simulink model "cosine_pow4"  (R2021b)
settings: Solver=VariableStepAuto  StartTime=0.0  StopTime=1  RelTol=1e-3
libraries: dspsrcs4 x1
settings Model: Creator=baggo  LastModifiedBy=baggo

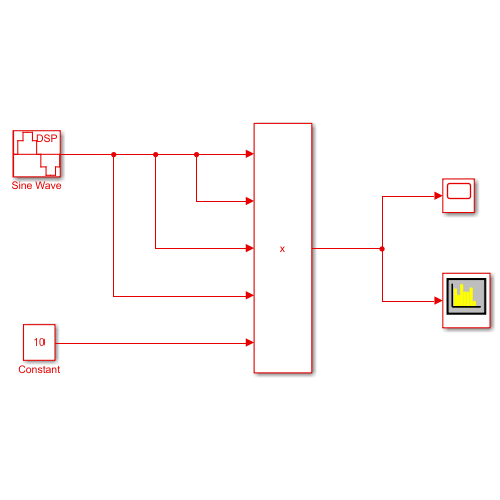
[thumbnail: Simulink's stored preview of the top-level diagram]
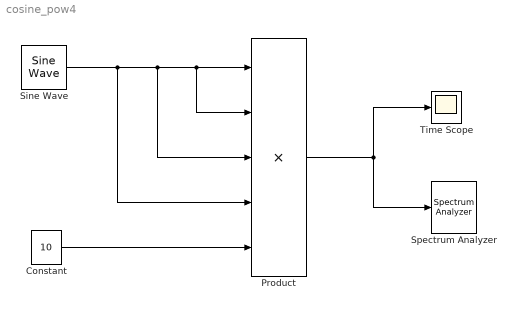
== system cosine_pow4 ==
  Constant : Constant  Value=10  VectorParams1D=off  SampleTime=-1
  Product : Product  Inputs=5
  Sine Wave : dspsrcs4/Sine Wave  Amplitude=1  Frequency=100e3  Phase=pi/2  SampleMode=Discrete  OutComplex=Real  CompMethod=Trigonometric fcn  TableSize=Speed  SampleTime=1/(4*1024e3)  SamplesPerFrame=1  ResetState=Restart at time zero  OutputFrames=off  dataType=double  wordLen=16  udDataType=sfix(16)  fracBitsMode=Best precision  numFracBits=15  OutDataTypeStr=double  LastOutDataTypeStr=double
  Spectrum Analyzer : SpectrumAnalyzer
  Time Scope : Scope
  wires:
  Sine Wave/1 -> Product/4, Product/3, Product/2, Product/1
  Constant/1 -> Product/5
  Product/1 -> Spectrum Analyzer/1, Time Scope/1
